simulink model "ProyectoAutomatasSimulink"  (R2015a)
settings: Solver=ode45  SolverMode=SingleTasking  StartTime=0.0  StopTime=90  RelTol=1e-3
values from neighbouring files (symbols this model uses):
  amaxh = 1    [ProyectoAutomatas.m]
  amaxt = 1    [ProyectoAutomatas.m]
  bah = Jh*nh*wposh    (= 1200355.55556)    [ProyectoAutomatas.m]
  bat = Jt*nt*wpost    (= 1966933.33333)    [ProyectoAutomatas.m]
  bh = beqh/Rd^2    (= 32)    [ProyectoAutomatas.m]
  bt = beqc/Rw^2    (= 120)    [ProyectoAutomatas.m]
  bw = 30*10^3    (= 30000)    [ProyectoAutomatas.m]
  dt = 0.001    [ProyectoAutomatas.m]
  g = 9.80665    [ProyectoAutomatas.m]
  Kisah = Ksah*wposh/nh    (= 150044444444)    [ProyectoAutomatas.m]
  Kisat = Ksat*wpost/nt    (= 245866666667)    [ProyectoAutomatas.m]
  Ksah = bah*wposh    (= 600177777.778)    [ProyectoAutomatas.m]
  Ksat = bat*wpost    (= 983466666.667)    [ProyectoAutomatas.m]
  Kw = 1800*10^3    (= 1800000)    [ProyectoAutomatas.m]
  lh0 = 5    [ProyectoAutomatas.m]
  mc = 50000    [ProyectoAutomatas.m]
  Mh = (Jdh+Jmh*rh^2)/Rd^2    (= 48014.2222222)    [ProyectoAutomatas.m]
  ml0 = 15000    [ProyectoAutomatas.m]
  mlempty = 17000    [ProyectoAutomatas.m]
  mlfull = 65000    [ProyectoAutomatas.m]
  Mt = mc+(Jwc+Jmc*rc^2)/Rw^2    (= 59008)    [ProyectoAutomatas.m]
  na = 3    [ProyectoAutomatas.m]
  rc = 15    [ProyectoAutomatas.m]
  Rd = 0.75    [ProyectoAutomatas.m]
  rh = 30    [ProyectoAutomatas.m]
  Rw = 0.5    [ProyectoAutomatas.m]
  Ttmax = ((Mt+mlfull)*amaxt+bt*vmaxt)*Rw/rc    (= 4149.6)    [ProyectoAutomatas.m]
  vh0 = 0    [ProyectoAutomatas.m]
  vlx0 = 0    [ProyectoAutomatas.m]
  vly0 = 0    [ProyectoAutomatas.m]
  vmaxh = 3    [ProyectoAutomatas.m]
  vmaxt = 4    [ProyectoAutomatas.m]
  vt0 = 0    [ProyectoAutomatas.m]
  xl0 = -30    [ProyectoAutomatas.m]
  xt0 = -30    [ProyectoAutomatas.m]
  yl0 = yt0-lh0-ml0*g/Kw    (= 39.9182779167)    [ProyectoAutomatas.m]
  yt0 = 45    [ProyectoAutomatas.m]
undefined symbols (not defined in the file or in its folder): sigbuilder_block
libraries: simulink x1
settings Model: Creator=Maxi Garcia  LastModifiedBy=Maxi Garcia
settings DataIOCC: SignalLoggingSaveFormat=ModelDataLogs
settings OptimizationCC: BlockReduction=off  BooleanDataType=off
settings DebuggingCC: SaveWithParameterizedLinksMsg=none  UnderspecifiedInitializationDetection=Classic  MergeDetectMultiDrivingBlocksExec=none  SignalResolutionControl=TryResolveAllWithWarning  MultiTaskDSMMsg=warning  MultiTaskCondExecSysMsg=none
settings HardwareCC: TargetUnknown=on

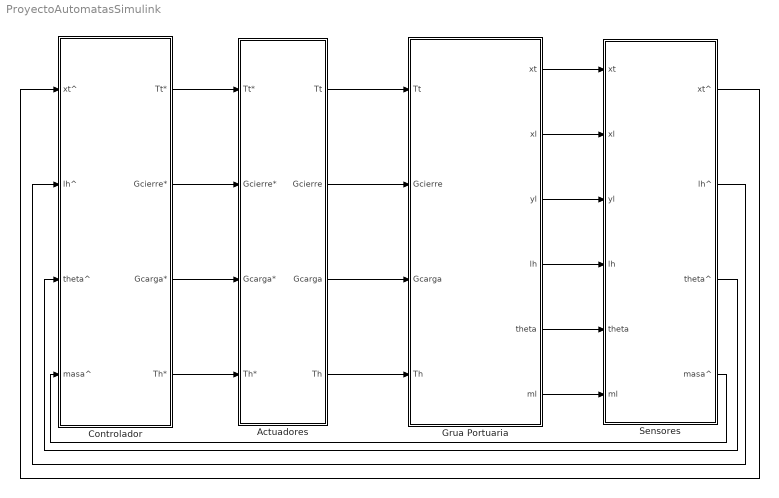
== system ProyectoAutomatasSimulink ==
  Actuadores : Subsystem
  Controlador : Subsystem
  Grua Portuaria : Subsystem
  Sensores : Subsystem
  wires:
  Grua Portuaria/1(xt) -> Sensores/1(xt)
  Grua Portuaria/4(lh) -> Sensores/4(lh)
  Grua Portuaria/5(theta) -> Sensores/5(theta)
  Actuadores/1(Tt) -> Grua Portuaria/1(Tt)
  Actuadores/2(Gcierre) -> Grua Portuaria/2(Gcierre)
  Actuadores/3(Gcarga) -> Grua Portuaria/3(Gcarga)
  Actuadores/4(Th) -> Grua Portuaria/4(Th)
  Controlador/1(Tt*) -> Actuadores/1(Tt*)
  Controlador/4(Th*) -> Actuadores/4(Th*)
  Controlador/2(Gcierre*) -> Actuadores/2(Gcierre*)
  Controlador/3(Gcarga*) -> Actuadores/3(Gcarga*)
  Sensores/3(theta^) -> Controlador/3(theta^)
  Sensores/2(lh^) -> Controlador/2(lh^)
  Sensores/1(xt^) -> Controlador/1(xt^)
  Grua Portuaria/6(ml) -> Sensores/6(ml)
  Grua Portuaria/2(xl) -> Sensores/2(xl)
  Grua Portuaria/3(yl) -> Sensores/3(yl)
  Sensores/4(masa^) -> Controlador/4(masa^)

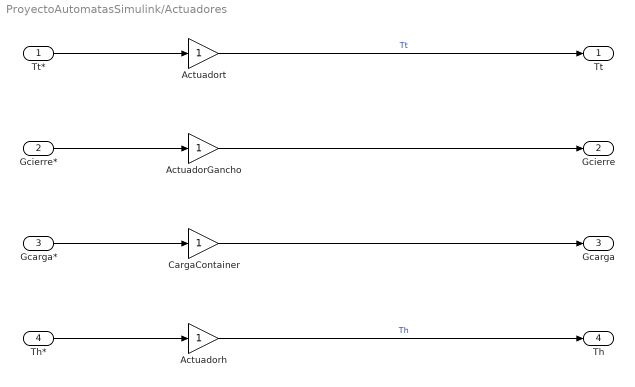
== system ProyectoAutomatasSimulink/Actuadores ==
  Tt* : Inport
  Gcierre* : Inport  Port=2
  Gcarga* : Inport  Port=3
  Th* : Inport  Port=4
  ActuadorGancho : Gain
  Actuadorh : Gain
  Actuadort : Gain
  CargaContainer : Gain
  Tt : Outport
  Gcierre : Outport  Port=2
  Gcarga : Outport  Port=3
  Th : Outport  Port=4
  wires:
  Th*/1 -> Actuadorh/1
  Actuadort/1 -> Tt/1  "Tt"
  Tt*/1 -> Actuadort/1
  ActuadorGancho/1 -> Gcierre/1
  CargaContainer/1 -> Gcarga/1
  Actuadorh/1 -> Th/1  "Th"
  Gcierre*/1 -> ActuadorGancho/1
  Gcarga*/1 -> CargaContainer/1

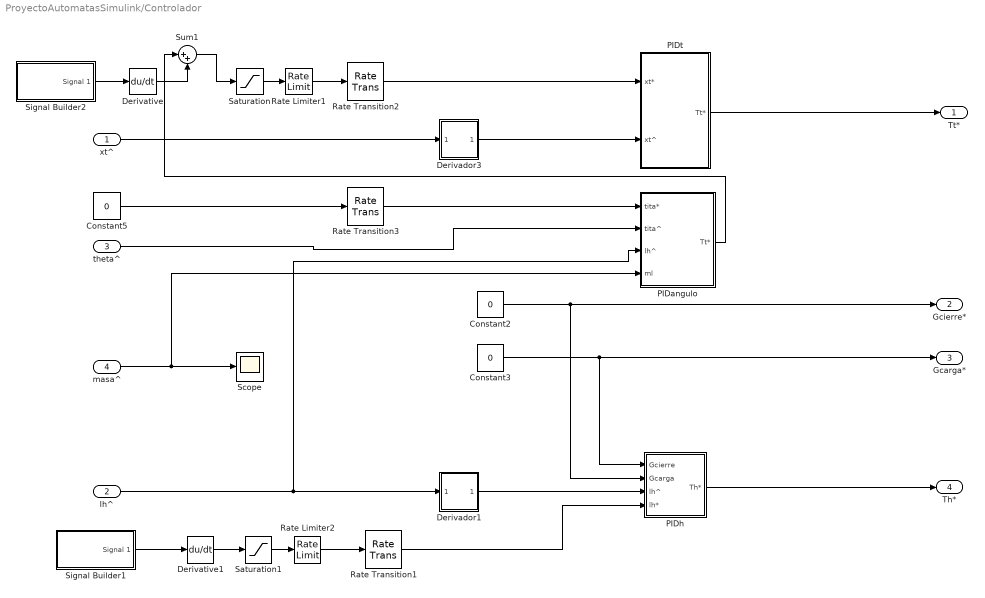
== system ProyectoAutomatasSimulink/Controlador ==
  xt^ : Inport
  lh^ : Inport  Port=2
  theta^ : Inport  Port=3
  masa^ : Inport  Port=4
  Constant2 : Constant  Value=0
  Constant3 : Constant  Value=0
  Constant5 : Constant  Value=0
  Derivador1 : Subsystem
  Derivador3 : Subsystem
  Derivative : Derivative
  Derivative1 : Derivative
  PIDangulo : Subsystem
  PIDh : Subsystem
  PIDt : Subsystem
  Rate Limiter1 : RateLimiter  RisingSlewLimit=amaxt  FallingSlewLimit=-amaxt  SampleTimeMode=inherited
  Rate Limiter2 : RateLimiter  RisingSlewLimit=amaxh  FallingSlewLimit=-amaxh  SampleTimeMode=inherited
  Rate Transition1 : RateTransition  X0=5  OutPortSampleTime=dt
  Rate Transition2 : RateTransition  OutPortSampleTime=dt
  Rate Transition3 : RateTransition  OutPortSampleTime=dt
  Saturation : Saturate  UpperLimit=vmaxt  LowerLimit=-vmaxt
  Saturation1 : Saturate  UpperLimit=vmaxh  LowerLimit=-vmaxh
  Scope : Scope
      settings: SaveName=ScopeData2
  Signal Builder1 : Subsystem  Tag=STV Subsys  LoadFcn=sigbuilder_block('load');  StartFcn=sigbuilder_block('start');  StopFcn=sigbuilder_block('stop');  ClipboardFcn=sigbuilder_block('clipboard');  mask(Sigbuilder block){}
      mask help: Simulink:masks:SigbuilderBlock_MD
      mask init:
      | if ~strcmp(get_param(bdroot(gcbh),'SimulationStatus'),'stopped') tuvar = sigbuilder_block('maskInit'); end
      settings: CopyFcn=sigbuilder_block('copy');  DeleteFcn=sigbuilder_block('delete');  ModelCloseFcn=sigbuilder_block('modelClose');  PreSaveFcn=sigbuilder_block('preSave');  PauseFcn=sigbuilder_block('pause');  ContinueFcn=sigbuilder_block('continue');  NameChangeFcn=sigbuilder_block('namechange');  OpenFcn=sigbuilder_block('open',[437.6 199.2 550.4 400 ]);  CloseFcn=sigbuilder_block('close');
      mask Display: plot(0, 0, 100, 100,[2, 2, 32, 32, 2], [68, 8, 8, 68, 68],[32, 2], [38, 38], [32, 19, 2],[53, 60, 44], [32, 17, 17, 2],[16, 16, 31, 31]);txt = getActiveGroup(gcbh);text(2, 100, txt,'verticalAlignment', 'top');
  Signal Builder2 : Subsystem  Tag=STV Subsys  LoadFcn=sigbuilder_block('load');  StartFcn=sigbuilder_block('start');  StopFcn=sigbuilder_block('stop');  ClipboardFcn=sigbuilder_block('clipboard');  mask(Sigbuilder block){}
      mask help: Simulink:masks:SigbuilderBlock_MD
      mask init:
      | if ~strcmp(get_param(bdroot(gcbh),'SimulationStatus'),'stopped') tuvar = sigbuilder_block('maskInit'); end
      settings: CopyFcn=sigbuilder_block('copy');  DeleteFcn=sigbuilder_block('delete');  ModelCloseFcn=sigbuilder_block('modelClose');  PreSaveFcn=sigbuilder_block('preSave');  PauseFcn=sigbuilder_block('pause');  ContinueFcn=sigbuilder_block('continue');  NameChangeFcn=sigbuilder_block('namechange');  OpenFcn=sigbuilder_block('open',[437.6 199.2 550.4 400 ]);  CloseFcn=sigbuilder_block('close');
      mask Display: plot(0, 0, 100, 100,[2, 2, 32, 32, 2], [68, 8, 8, 68, 68],[32, 2], [38, 38], [32, 19, 2],[53, 60, 44], [32, 17, 17, 2],[16, 16, 31, 31]);txt = getActiveGroup(gcbh);text(2, 100, txt,'verticalAlignment', 'top');
  Sum1 : Sum  Inputs=|++
  Tt* : Outport
  Gcierre* : Outport  Port=2
  Gcarga* : Outport  Port=3
  Th* : Outport  Port=4
  wires:
  Constant2/1 -> PIDh/2(Gcarga), Gcierre*/1
  Constant3/1 -> PIDh/1(Gcierre), Gcarga*/1
  PIDh/1(Th*) -> Th*/1
  xt^/1 -> Derivador3/1(In1)
  Signal Builder2/1(Signal 1) -> Derivative/1
  Constant5/1 -> Rate Transition3/1
  lh^/1 -> PIDangulo/3(lh^), Derivador1/1(In1)
  Derivador1/1(Out1) -> PIDh/3(lh^)
  Derivador3/1(Out1) -> PIDt/2(xt^)
  masa^/1 -> PIDangulo/4(ml), Scope/1
  theta^/1 -> PIDangulo/2(tita^)
  Rate Transition3/1 -> PIDangulo/1(tita*)
  PIDt/1(Tt*) -> Tt*/1
  Rate Transition1/1 -> PIDh/4(lh*)
  Rate Transition2/1 -> PIDt/1(xt*)
  Rate Limiter1/1 -> Rate Transition2/1
  Derivative/1 -> Sum1/2
  Saturation/1 -> Rate Limiter1/1
  Derivative1/1 -> Saturation1/1
  Saturation1/1 -> Rate Limiter2/1
  Rate Limiter2/1 -> Rate Transition1/1
  Signal Builder1/1(Signal 1) -> Derivative1/1
  Sum1/1 -> Saturation/1
  PIDangulo/1(Tt*) -> Sum1/1

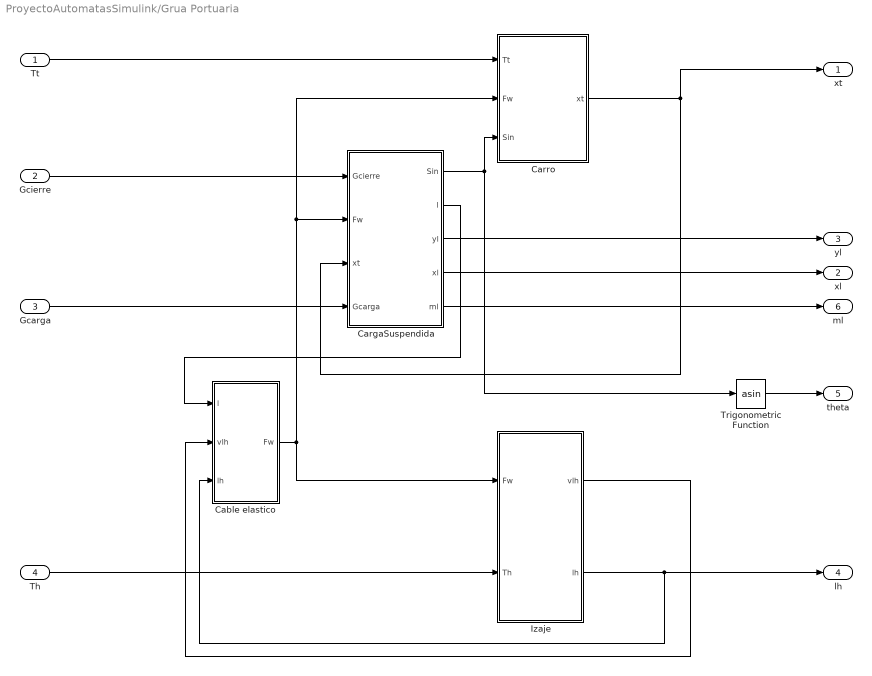
== system ProyectoAutomatasSimulink/Grua Portuaria ==
  Tt : Inport
  Gcierre : Inport  Port=2
  Gcarga : Inport  Port=3
  Th : Inport  Port=4
  Cable elastico : Subsystem
  CargaSuspendida : Subsystem
  Carro : Subsystem
  Izaje : Subsystem
  Trigonometric Function : Trigonometry  Operator=asin
  xt : Outport
  xl : Outport  Port=2
  yl : Outport  Port=3
  lh : Outport  Port=4
  theta : Outport  Port=5
  ml : Outport  Port=6
  wires:
  Izaje/1(vlh) -> Cable elastico/2(vlh)
  CargaSuspendida/1(Sin) -> Carro/3(Sin), Trigonometric Function/1
  Th/1 -> Izaje/2(Th)
  Izaje/2(lh) -> Cable elastico/3(lh), lh/1
  Carro/1(xt) -> xt/1, CargaSuspendida/3(xt)
  Gcierre/1 -> CargaSuspendida/1(Gcierre)
  Gcarga/1 -> CargaSuspendida/4(Gcarga)
  Tt/1 -> Carro/1(Tt)
  CargaSuspendida/2(l) -> Cable elastico/1(l)
  Cable elastico/1(Fw) -> Izaje/1(Fw), Carro/2(Fw), CargaSuspendida/2(Fw)
  Trigonometric Function/1 -> theta/1
  CargaSuspendida/5(ml) -> ml/1
  CargaSuspendida/4(xl) -> xl/1
  CargaSuspendida/3(yl) -> yl/1

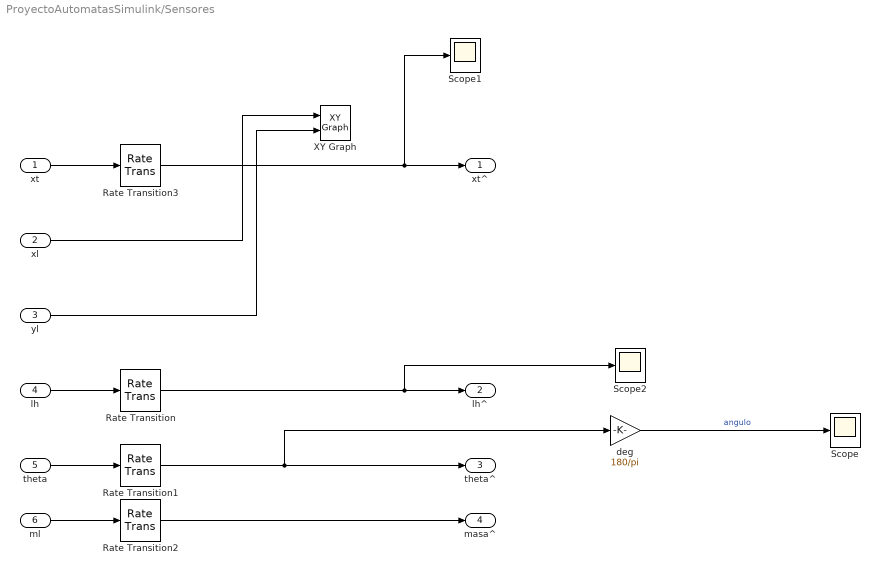
== system ProyectoAutomatasSimulink/Sensores ==
  xt : Inport
  xl : Inport  Port=2
  yl : Inport  Port=3
  lh : Inport  Port=4
  theta : Inport  Port=5
  ml : Inport  Port=6
  Rate Transition : RateTransition  X0=5  OutPortSampleTime=dt
  Rate Transition1 : RateTransition  OutPortSampleTime=dt
  Rate Transition2 : RateTransition  X0=ml0  OutPortSampleTime=dt
  Rate Transition3 : RateTransition  X0=-30  OutPortSampleTime=dt
  Scope : Scope
      settings: YMin=-90  YMax=90
  Scope1 : Scope
      settings: YMin=72.5  YMax=97.5
  Scope2 : Scope
      settings: YMin=39.2  YMax=39.85  SaveName=ScopeData8
  XY Graph : simulink/Sinks/XY Graph  xmin=-35  xmax=55  ymin=-25  ymax=45  st=-1
  deg : Gain  Gain=180/pi
  xt^ : Outport
  lh^ : Outport  Port=2
  theta^ : Outport  Port=3
  masa^ : Outport  Port=4
  wires:
  theta/1 -> Rate Transition1/1
  yl/1 -> XY Graph/2
  xl/1 -> XY Graph/1
  xt/1 -> Rate Transition3/1
  Rate Transition1/1 -> deg/1, theta^/1
  deg/1 -> Scope/1  "angulo"
  Rate Transition2/1 -> masa^/1
  ml/1 -> Rate Transition2/1
  lh/1 -> Rate Transition/1
  Rate Transition/1 -> Scope2/1, lh^/1
  Rate Transition3/1 -> Scope1/1, xt^/1

== system ProyectoAutomatasSimulink/Controlador/Derivador1 ==
  In1 : Inport
  1/dt : Gain  Gain=1/dt
  Delay3 : Delay  DelayLength=1  InitialCondition=5  SampleTime=dt
  Sum6 : Sum  Inputs=|+-
  Out1 : Outport
  wires:
  In1/1 -> Delay3/1, Sum6/1
  Delay3/1 -> Sum6/2
  Sum6/1 -> 1/dt/1
  1/dt/1 -> Out1/1

== system ProyectoAutomatasSimulink/Controlador/Derivador3 ==
  In1 : Inport
  1/dt : Gain  Gain=1/dt
  Delay3 : Delay  DelayLength=1  InitialCondition=-30  SampleTime=dt
  Sum6 : Sum  Inputs=|+-
  Out1 : Outport
  wires:
  In1/1 -> Delay3/1, Sum6/1
  Delay3/1 -> Sum6/2
  Sum6/1 -> 1/dt/1
  1/dt/1 -> Out1/1

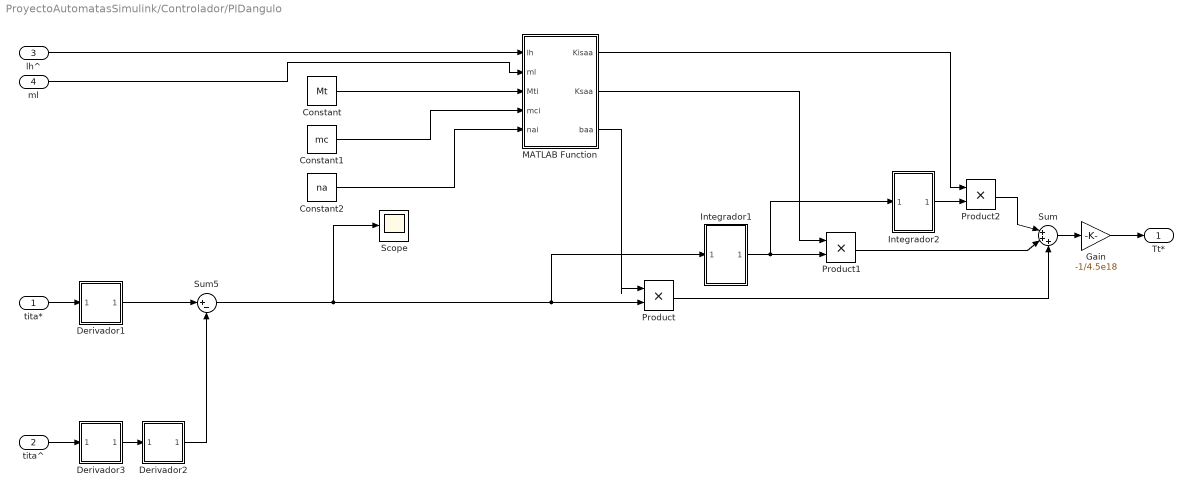
== system ProyectoAutomatasSimulink/Controlador/PIDangulo ==
  tita* : Inport
  tita^ : Inport  Port=2
  lh^ : Inport  Port=3
  ml : Inport  Port=4
  Constant : Constant  Value=Mt
  Constant1 : Constant  Value=mc
  Constant2 : Constant  Value=na
  Derivador1 : Subsystem
  Derivador2 : Subsystem
  Derivador3 : Subsystem
  Gain : Gain  Gain=-1/4.5e18
  Integrador1 : Subsystem
  Integrador2 : Subsystem
  MATLAB Function : MATLAB Function  TreatAsAtomicUnit=on
  Product : Product
  Product1 : Product
  Product2 : Product
  Scope : Scope
      settings: YMin=-1.2  YMax=0.7  SaveName=ScopeData9
  Sum : Sum  Inputs=|+++
  Sum5 : Sum  Inputs=|+-
  Tt* : Outport
  wires:
  tita*/1 -> Derivador1/1(In1)
  lh^/1 -> MATLAB Function/1(lh)
  Sum/1 -> Gain/1
  Product/1 -> Sum/3
  Integrador1/1(Out1) -> Integrador2/1(In1), Product1/2
  Product1/1 -> Sum/2
  Integrador2/1(Out1) -> Product2/2
  tita^/1 -> Derivador3/1(In1)
  Sum5/1 -> Scope/1, Integrador1/1(In1), Product/2
  MATLAB Function/3(baa) -> Product/1
  MATLAB Function/2(Ksaa) -> Product1/1
  MATLAB Function/1(Kisaa) -> Product2/1
  ml/1 -> MATLAB Function/2(ml)
  Constant/1 -> MATLAB Function/3(Mti)
  Constant1/1 -> MATLAB Function/4(mci)
  Constant2/1 -> MATLAB Function/5(nai)
  Derivador3/1(Out1) -> Derivador2/1(In1)
  Derivador1/1(Out1) -> Sum5/1
  Gain/1 -> Tt*/1
  Product2/1 -> Sum/1
  Derivador2/1(Out1) -> Sum5/2

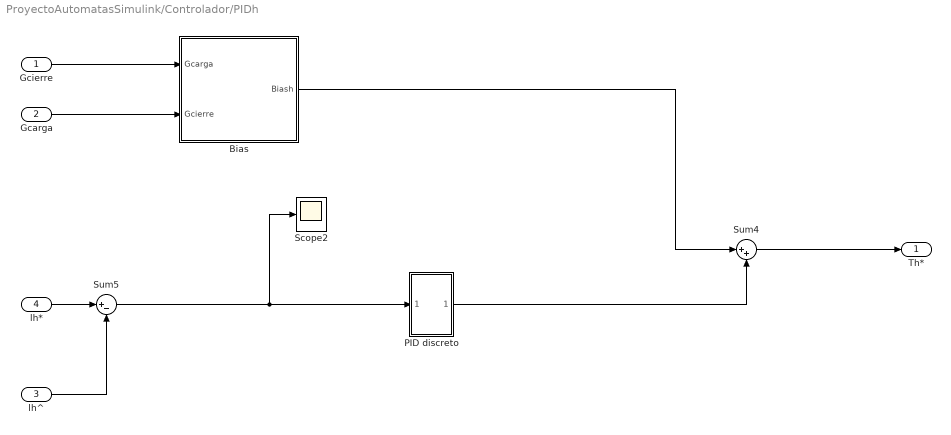
== system ProyectoAutomatasSimulink/Controlador/PIDh ==
  Gcierre : Inport
  Gcarga : Inport  Port=2
  lh^ : Inport  Port=3
  lh* : Inport  Port=4
  Bias : Subsystem
  PID discreto : Subsystem
  Scope2 : Scope
      settings: TimeRange=80  YMin=-3e+24  YMax=6e+24  SaveName=ScopeData6
  Sum4 : Sum  Inputs=|++
  Sum5 : Sum  Inputs=|+-
  Th* : Outport
  wires:
  Bias/1(Biash) -> Sum4/1
  Gcierre/1 -> Bias/1(Gcarga)
  Gcarga/1 -> Bias/2(Gcierre)
  Sum4/1 -> Th*/1
  lh*/1 -> Sum5/1
  lh^/1 -> Sum5/2
  PID discreto/1(Out1) -> Sum4/2
  Sum5/1 -> PID discreto/1(In1), Scope2/1

== system ProyectoAutomatasSimulink/Controlador/PIDt ==
  xt* : Inport
  xt^ : Inport  Port=2
  PID discreto : Subsystem
  Scope : Scope
      settings: YMin=-0.0004  YMax=0.0009  SaveName=ScopeData7
  Sum5 : Sum  Inputs=|+-
  Tt* : Outport
  wires:
  xt*/1 -> Sum5/1
  xt^/1 -> Sum5/2
  Sum5/1 -> Scope/1, PID discreto/1(In1)
  PID discreto/1(Out1) -> Tt*/1

== system ProyectoAutomatasSimulink/Controlador/Signal Builder1 ==
  Demux : Demux  Tag=STV Demux  Outputs=1
  FromWs : FromWorkspace  Tag=STV FromWs  VariableName=tuvar  SampleTime=0
      SigBuilderData=|
      | common.afterFinalStr = 'Extrapolate'
      | common.sampleTime = 0
      | dataSet.timeRange = [0 80]
      | dataSet.name = 'Group 1'
      | sbobj.Groups.Name = 'Group 1'
      | sbobj.Groups.Signals.Name = 'Signal 1'
      | sbobj.Groups.Signals.XData = [0 2 37 39 74 80]
      | sbobj.Groups.Signals.YData = [5 5 40 40 5 5]
      | sbobj.Groups.TimeRange = [0 80]
  Signal 1 : Outport  Tag=STV Outport
  wires:
  Demux/1 -> Signal 1/1
  FromWs/1 -> Demux/1

== system ProyectoAutomatasSimulink/Controlador/Signal Builder2 ==
  Demux : Demux  Tag=STV Demux  Outputs=1
  FromWs : FromWorkspace  Tag=STV FromWs  VariableName=tuvar  SampleTime=0
      SigBuilderData=|
      | common.afterFinalStr = 'Extrapolate'
      | common.sampleTime = 0
      | dataSet.timeRange = [0 80]
      | dataSet.name = 'Group 1'
      | sbobj.Groups.Name = 'Group 1'
      | sbobj.Groups.Signals.Name = 'Signal 1'
      | sbobj.Groups.Signals.XData = [0 2 37 39 74 80]
      | sbobj.Groups.Signals.YData = [-30 -30 50 50 -30 -30]
      | sbobj.Groups.TimeRange = [0 80]
  Signal 1 : Outport  Tag=STV Outport
  wires:
  Demux/1 -> Signal 1/1
  FromWs/1 -> Demux/1

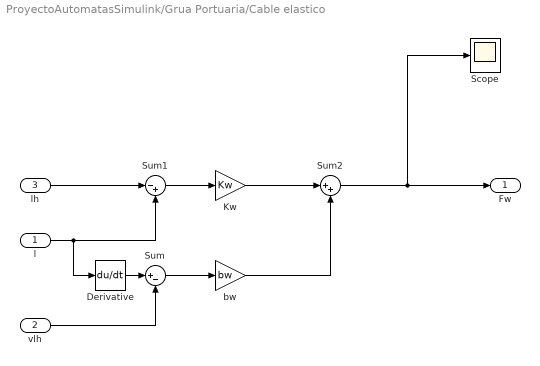
== system ProyectoAutomatasSimulink/Grua Portuaria/Cable elastico ==
  l : Inport
  vlh : Inport  Port=2
  lh : Inport  Port=3
  Derivative : Derivative
  Kw : Gain  Gain=Kw
  Scope : Scope
      settings: YMin=-90  YMax=0  SaveName=ScopeData3
  Sum : Sum  Inputs=|+-
  Sum1 : Sum  Inputs=|-+
  Sum2 : Sum  Inputs=|++
  bw : Gain  Gain=bw
  Fw : Outport
  wires:
  l/1 -> Derivative/1, Sum1/2
  Derivative/1 -> Sum/1
  vlh/1 -> Sum/2
  Sum1/1 -> Kw/1
  Sum/1 -> bw/1
  Kw/1 -> Sum2/1
  bw/1 -> Sum2/2
  Sum2/1 -> Scope/1, Fw/1
  lh/1 -> Sum1/1

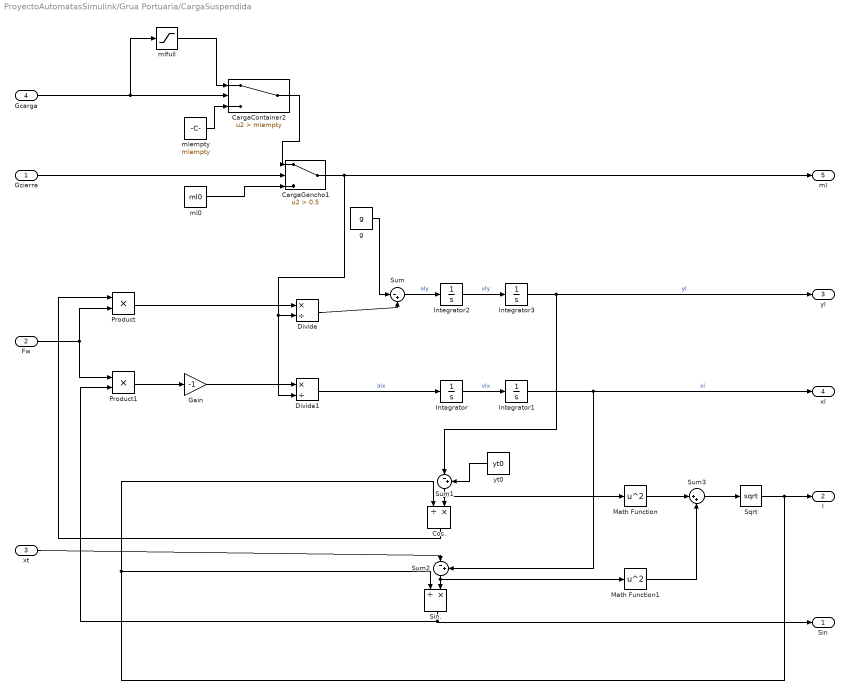
== system ProyectoAutomatasSimulink/Grua Portuaria/CargaSuspendida ==
  Gcierre : Inport
  Fw : Inport  Port=2
  xt : Inport  Port=3
  Gcarga : Inport  Port=4
  CargaContainer2 : Switch  Criteria=u2 > Threshold  Threshold=mlempty
  CargaGancho1 : Switch  Criteria=u2 > Threshold  Threshold=0.5
  Cos. : Product  Inputs=/*
  Divide : Product  Inputs=*/
  Divide1 : Product  Inputs=*/
  Gain : Gain  Gain=-1
  Integrator : Integrator  InitialCondition=vlx0
  Integrator1 : Integrator  InitialCondition=xl0
  Integrator2 : Integrator  InitialCondition=vly0
  Integrator3 : Integrator  InitialCondition=yl0
  Math Function : Math  Operator=square  SaturateOnIntegerOverflow=on
  Math Function1 : Math  Operator=square  SaturateOnIntegerOverflow=on
  Product : Product
  Product1 : Product
  Sin. : Product  Inputs=/*
  Sqrt : Sqrt  SaturateOnIntegerOverflow=on
  Sum : Sum  Inputs=|-+
  Sum1 : Sum  Inputs=|-+
  Sum2 : Sum  Inputs=|-+
  Sum3 : Sum  Inputs=|++
  g : Constant  Value=g
  "ml0 " : Constant  Value=ml0
  mlempty : Constant  Value=mlempty
  "mlfull " : Saturate  UpperLimit=mlfull  LowerLimit=-Ttmax
  yt0 : Constant  Value=yt0
  Sin : Outport
  l : Outport  Port=2
  yl : Outport  Port=3
  xl : Outport  Port=4
  ml : Outport  Port=5
  wires:
  CargaGancho1/1 -> ml/1, Divide/2, Divide1/2
  Gcierre/1 -> CargaGancho1/2
  Fw/1 -> Product1/1, Product/2
  Product/1 -> Divide/1
  Product1/1 -> Gain/1
  Gain/1 -> Divide1/1
  Divide/1 -> Sum/2
  g/1 -> Sum/1
  Integrator/1 -> Integrator1/1  "vlx"
  Integrator1/1 -> xl/1, Sum2/2  "xl"
  Integrator2/1 -> Integrator3/1  "vly"
  Sum1/1 -> Cos./2, Math Function/1
  yt0/1 -> Sum1/2
  Integrator3/1 -> Sum1/1, yl/1  "yl"
  Cos./1 -> Product/1
  Sum2/1 -> Math Function1/1, Sin./2
  xt/1 -> Sum2/1
  Sin./1 -> Sin/1, Product1/2
  Math Function/1 -> Sum3/1
  Math Function1/1 -> Sum3/2
  Sum3/1 -> Sqrt/1
  CargaContainer2/1 -> CargaGancho1/1
  Gcarga/1 -> "mlfull "/1, CargaContainer2/2
  "ml0 "/1 -> CargaGancho1/3
  mlempty/1 -> CargaContainer2/3
  "mlfull "/1 -> CargaContainer2/1
  Sqrt/1 -> Cos./1, Sin./1, l/1
  Sum/1 -> Integrator2/1  "aly"
  Divide1/1 -> Integrator/1  "alx"

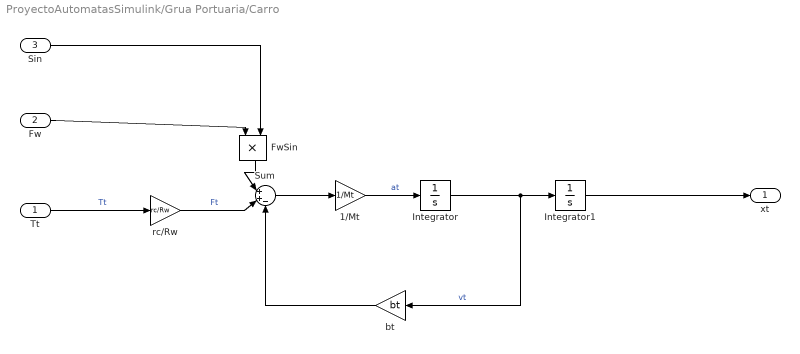
== system ProyectoAutomatasSimulink/Grua Portuaria/Carro ==
  Tt : Inport
  Fw : Inport  Port=2
  Sin : Inport  Port=3
  1/Mt : Gain  Gain=1/Mt
  FwSin : Product
  Integrator : Integrator  InitialCondition=vt0
  Integrator1 : Integrator  InitialCondition=xt0
  Sum : Sum  Inputs=|++-
  bt : Gain  Gain=bt
  rc/Rw : Gain  Gain=rc/Rw
  xt : Outport
  wires:
  Integrator1/1 -> xt/1
  rc/Rw/1 -> Sum/2  "Ft"
  Tt/1 -> rc/Rw/1  "Tt"
  1/Mt/1 -> Integrator/1  "at"
  bt/1 -> Sum/3
  Sum/1 -> 1/Mt/1
  Integrator/1 -> bt/1, Integrator1/1  "vt"
  Sin/1 -> FwSin/2
  FwSin/1 -> Sum/1
  Fw/1 -> FwSin/1

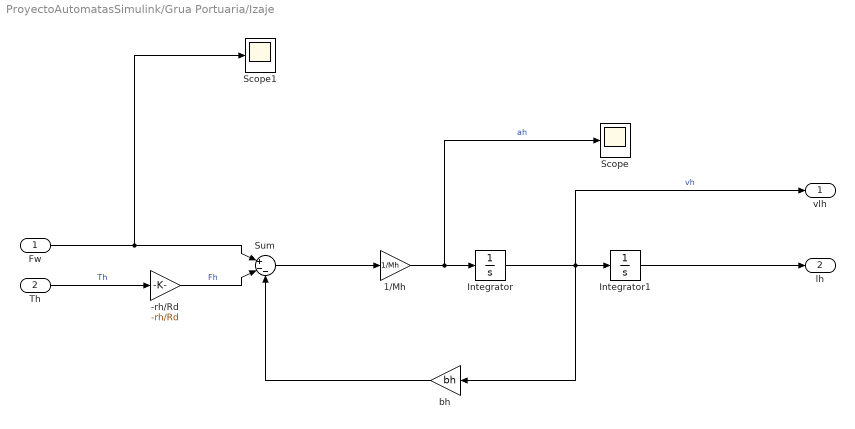
== system ProyectoAutomatasSimulink/Grua Portuaria/Izaje ==
  Fw : Inport
  Th : Inport  Port=2
  "-rh/Rd\t" : Gain  Gain=-rh/Rd
  1/Mh : Gain  Gain=1/Mh
  Integrator : Integrator  InitialCondition=vh0
  Integrator1 : Integrator  InitialCondition=lh0
  Scope : Scope
      settings: YMin=-90  YMax=0  SaveName=ScopeData4
  Scope1 : Scope
      settings: YMin=-90  YMax=0  SaveName=ScopeData5
  Sum : Sum  Inputs=|+--
  bh : Gain  Gain=bh
  vlh : Outport
  lh : Outport  Port=2
  wires:
  Integrator1/1 -> lh/1
  "-rh/Rd\t"/1 -> Sum/2  "Fh"
  Th/1 -> "-rh/Rd\t"/1  "Th"
  1/Mh/1 -> Scope/1, Integrator/1  "ah"
  bh/1 -> Sum/3
  Sum/1 -> 1/Mh/1
  Integrator/1 -> vlh/1, bh/1, Integrator1/1  "vh"
  Fw/1 -> Scope1/1, Sum/1

== system ProyectoAutomatasSimulink/Controlador/PIDangulo/Derivador1 ==
  In1 : Inport
  1/dt : Gain  Gain=1/dt
  Delay3 : Delay  DelayLength=1  InitialCondition=0  SampleTime=dt
  Sum6 : Sum  Inputs=|+-
  Out1 : Outport
  wires:
  In1/1 -> Delay3/1, Sum6/1
  Delay3/1 -> Sum6/2
  Sum6/1 -> 1/dt/1
  1/dt/1 -> Out1/1

== system ProyectoAutomatasSimulink/Controlador/PIDangulo/Derivador2 ==
  In1 : Inport
  1/dt : Gain  Gain=1/dt
  Delay3 : Delay  DelayLength=1  InitialCondition=0  SampleTime=dt
  Sum6 : Sum  Inputs=|+-
  Out1 : Outport
  wires:
  In1/1 -> Delay3/1, Sum6/1
  Delay3/1 -> Sum6/2
  Sum6/1 -> 1/dt/1
  1/dt/1 -> Out1/1

== system ProyectoAutomatasSimulink/Controlador/PIDangulo/Derivador3 ==
  In1 : Inport
  1/dt : Gain  Gain=1/dt
  Delay3 : Delay  DelayLength=1  InitialCondition=0  SampleTime=dt
  Sum6 : Sum  Inputs=|+-
  Out1 : Outport
  wires:
  In1/1 -> Delay3/1, Sum6/1
  Delay3/1 -> Sum6/2
  Sum6/1 -> 1/dt/1
  1/dt/1 -> Out1/1

== system ProyectoAutomatasSimulink/Controlador/PIDangulo/Integrador1 ==
  In1 : Inport
  Delay3 : Delay  DelayLength=1  SampleTime=dt
  Sum6 : Sum  Inputs=|++
  dt : Gain  Gain=dt
  Out1 : Outport
  wires:
  Delay3/1 -> Sum6/2
  Sum6/1 -> Out1/1, Delay3/1
  dt/1 -> Sum6/1
  In1/1 -> dt/1

== system ProyectoAutomatasSimulink/Controlador/PIDangulo/Integrador2 ==
  In1 : Inport
  Delay3 : Delay  DelayLength=1  SampleTime=dt
  Sum6 : Sum  Inputs=|++
  dt : Gain  Gain=dt
  Out1 : Outport
  wires:
  Delay3/1 -> Sum6/2
  Sum6/1 -> Out1/1, Delay3/1
  dt/1 -> Sum6/1
  In1/1 -> dt/1

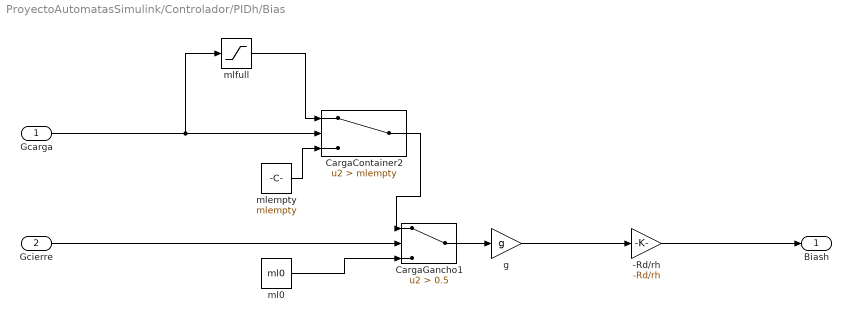
== system ProyectoAutomatasSimulink/Controlador/PIDh/Bias ==
  Gcarga : Inport
  Gcierre : Inport  Port=2
  -Rd/rh : Gain  Gain=-Rd/rh
  CargaContainer2 : Switch  Criteria=u2 > Threshold  Threshold=mlempty
  CargaGancho1 : Switch  Criteria=u2 > Threshold  Threshold=0.5
  g : Gain  Gain=g
  "ml0 " : Constant  Value=ml0
  mlempty : Constant  Value=mlempty
  "mlfull " : Saturate  UpperLimit=mlfull  LowerLimit=-Ttmax
  Biash : Outport
  wires:
  Gcarga/1 -> "mlfull "/1, CargaContainer2/2
  CargaContainer2/1 -> CargaGancho1/1
  mlempty/1 -> CargaContainer2/3
  Gcierre/1 -> CargaGancho1/2
  "ml0 "/1 -> CargaGancho1/3
  "mlfull "/1 -> CargaContainer2/1
  CargaGancho1/1 -> g/1
  g/1 -> -Rd/rh/1
  -Rd/rh/1 -> Biash/1

== system ProyectoAutomatasSimulink/Controlador/PIDh/PID discreto ==
  In1 : Inport
  Integrador : Subsystem
  Integrador1 : Subsystem
  Kisah : Gain  Gain=Kisah
  Ksah : Gain  Gain=Ksah
  Sum : Sum  Inputs=|+++
  bah : Gain  Gain=bah
  Out1 : Outport
  wires:
  In1/1 -> Integrador1/1(In1), bah/1
  bah/1 -> Sum/3
  Sum/1 -> Out1/1
  Ksah/1 -> Sum/2
  Kisah/1 -> Sum/1
  Integrador/1(Out1) -> Kisah/1
  Integrador1/1(Out1) -> Integrador/1(In1), Ksah/1

== system ProyectoAutomatasSimulink/Controlador/PIDt/PID discreto ==
  In1 : Inport
  Integrador : Subsystem
  Integrador1 : Subsystem
  Kisat : Gain  Gain=Kisat
  Ksat : Gain  Gain=Ksat
  Sum : Sum  Inputs=|+++
  bat : Gain  Gain=bat
  Out1 : Outport
  wires:
  bat/1 -> Sum/3
  Ksat/1 -> Sum/2
  Kisat/1 -> Sum/1
  Sum/1 -> Out1/1
  In1/1 -> Integrador1/1(In1), bat/1
  Integrador/1(Out1) -> Kisat/1
  Integrador1/1(Out1) -> Integrador/1(In1), Ksat/1

== system ProyectoAutomatasSimulink/Controlador/PIDh/PID discreto/Integrador ==
  In1 : Inport
  Delay3 : Delay  DelayLength=1  SampleTime=dt
  Sum6 : Sum  Inputs=|++
  dt : Gain  Gain=dt
  Out1 : Outport
  wires:
  Delay3/1 -> Sum6/2
  Sum6/1 -> Out1/1, Delay3/1
  dt/1 -> Sum6/1
  In1/1 -> dt/1

== system ProyectoAutomatasSimulink/Controlador/PIDh/PID discreto/Integrador1 ==
  In1 : Inport
  Delay3 : Delay  DelayLength=1  SampleTime=dt
  Sum6 : Sum  Inputs=|++
  dt : Gain  Gain=dt
  Out1 : Outport
  wires:
  Delay3/1 -> Sum6/2
  Sum6/1 -> Out1/1, Delay3/1
  dt/1 -> Sum6/1
  In1/1 -> dt/1

== system ProyectoAutomatasSimulink/Controlador/PIDt/PID discreto/Integrador ==
  In1 : Inport
  Delay3 : Delay  DelayLength=1  SampleTime=dt
  Sum6 : Sum  Inputs=|++
  dt : Gain  Gain=dt
  Out1 : Outport
  wires:
  Delay3/1 -> Sum6/2
  Sum6/1 -> Out1/1, Delay3/1
  dt/1 -> Sum6/1
  In1/1 -> dt/1

== system ProyectoAutomatasSimulink/Controlador/PIDt/PID discreto/Integrador1 ==
  In1 : Inport
  Delay3 : Delay  DelayLength=1  SampleTime=dt
  Sum6 : Sum  Inputs=|++
  dt : Gain  Gain=dt
  Out1 : Outport
  wires:
  Delay3/1 -> Sum6/2
  Sum6/1 -> Out1/1, Delay3/1
  dt/1 -> Sum6/1
  In1/1 -> dt/1

== matlab function ProyectoAutomatasSimulink/Controlador/PIDangulo/MATLAB Function ==
  data: Kisaa output; Ksaa output; baa output; lh input; ml input; Mti input; mci input; nai input
function [Kisaa,Ksaa,baa]= fcn(lh,ml,Mti,mci,nai)

persistent Mt
if isempty(Mt)
   Mt=Mti;
end
persistent mc
if isempty(mc)
   mc=mci;
end
persistent na
if isempty(na)
   na=nai;
end
persistent g
if isempty(g)
   g=9.80665;
end

Ma=(ml+Mt)/(mc+ml)*lh;                     %debe multiplicarsele el lh
wa=(4*(Mt+ml)*Mt*g)/(2*(Mt+ml))*lh^-0.5;        %debe multiplicarsele el lh^-0.5
wposa=10*wa;
baa=Ma*na*wposa;
Ksaa=baa*wposa;
Kisaa=Ksaa*wposa/na;
